simulink model "WaterDistSystem"  (R2023b)
settings: Solver=VariableStepAuto  StartTime=0.0  StopTime=inf  RelTol=1e-3
InitFcn:
  | seedGenerator
undefined symbols (not defined in the file or in its folder): hMin, maxCost, maxRep1, maxRep2, maxRep3, maxSteps, maxTime, meanFail1, meanFail2, meanFail3, minRep1, minRep2, minRep3, PenaltyCost, PenaltyPerformance, PenaltyResilience, PenaltySafety, RewardCost, RewardPerformance, RewardResilience, RewardSafety, rngSeed, singleReward, supCheck, supDeg, supFull, supNo, varFail1, varFail2, varFail3
libraries: simulink x4, rllib x1
settings Model: NumberOfSteps=10  SnapshotBufferSize=50  SnapshotInterval=50  Creator=sebru  LastModifiedBy=juliu
settings OptimizationCC: DefaultParameterBehavior=Inlined  EnhancedBackFolding=on  PassReuseOutputArgsAs=Individual arguments  ZeroExternalMemoryAtStartup=off  ZeroInternalMemoryAtStartup=off  OptimizeBlockOrder=speed  DifferentSizesBufferReuse=on  OptimizationCustomize=off  EfficientTunableParamExpr=on
settings DebuggingCC: AlgebraicLoopMsg=error  ParameterTunabilityLossMsg=error
settings ModelReferenceCC: EnableRefExpFcnMdlSchedulingChecks=on
settings SFSimCC: MATLABDynamicMemAlloc=off
settings RTWCC: Description=Embedded Coder  SystemTargetFile=ert.tlc  TemplateMakefile=ert_default_tmf
settings CodeAppCC: ForceParamTrailComments=on  IgnoreCustomStorageClasses=off  OperatorAnnotations=on  SimulinkDataObjDesc=on  SFDataObjDesc=on  InsertBlockDesc=on
settings ERTTargetCC: TargetLangStandard=C99 (ISO)  GenerateSampleERTMain=on  InlinedParameterPlacement=NonHierarchical  ERTCustomFileTemplate=example_file_process.tlc

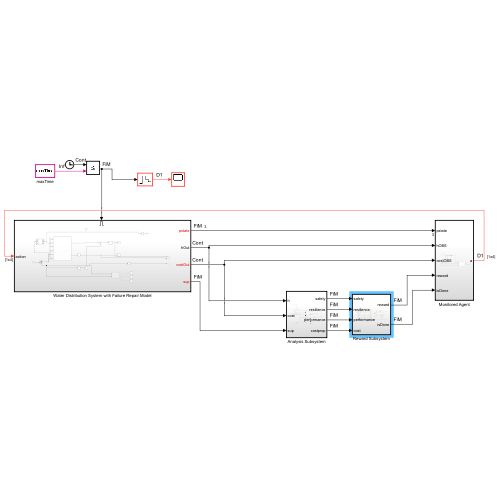
[thumbnail: Simulink's stored preview of the top-level diagram]
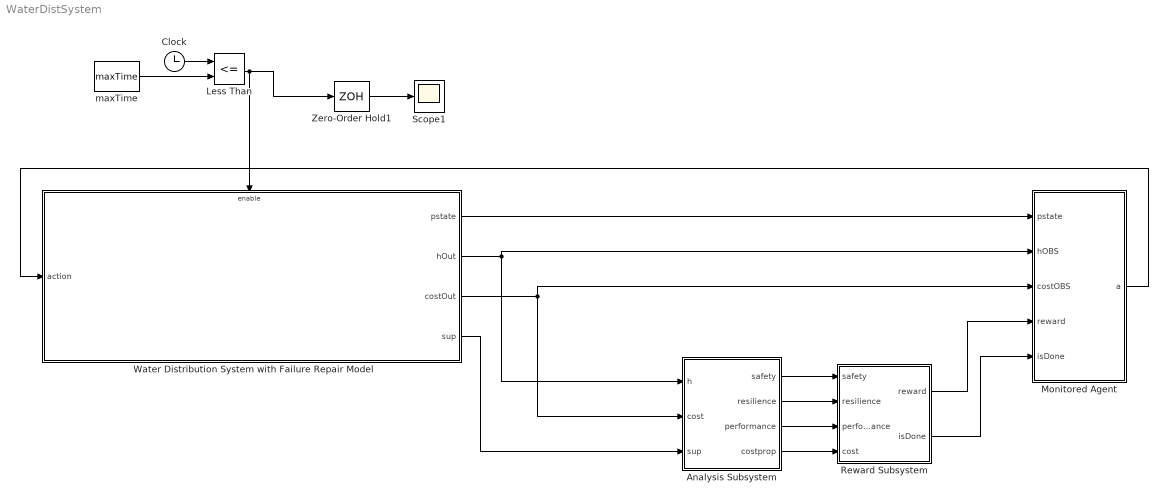
== system WaterDistSystem ==
  Analysis Subsystem : Subsystem
  Clock : Clock
  Less Than : RelationalOperator  Operator=<=  OutDataTypeStr=boolean  RndMeth=Simplest  InputSameDT=off
  Monitored Agent : Subsystem
  Reward Subsystem : Subsystem
  Scope1 : Scope
  Water Distribution System with Failure Repair Model : Subsystem  TreatAsAtomicUnit=on
      settings: MinAlgLoopOccurrences=on
  Zero-Order Hold1 : ZeroOrderHold  SampleTime=-1
  maxTime : Constant  Value=maxTime
  wires:
  Clock/1 -> Less Than/1
  Less Than/1 -> Zero-Order Hold1/1, Water Distribution System with Failure Repair Model/Enable
  maxTime/1 -> Less Than/2
  Monitored Agent/1(a) -> Water Distribution System with Failure Repair Model/1(action)
  Water Distribution System with Failure Repair Model/2(hOut) -> Analysis Subsystem/1(h), Monitored Agent/2(hOBS)
  Water Distribution System with Failure Repair Model/3(costOut) -> Analysis Subsystem/2(cost), Monitored Agent/3(costOBS)
  Water Distribution System with Failure Repair Model/1(pstate) -> Monitored Agent/1(pstate)
  Reward Subsystem/1(reward) -> Monitored Agent/4(reward)
  Reward Subsystem/2(isDone) -> Monitored Agent/5(isDone)
  Water Distribution System with Failure Repair Model/4(sup) -> Analysis Subsystem/3(sup)
  Zero-Order Hold1/1 -> Scope1/1
  Analysis Subsystem/2(resilience) -> Reward Subsystem/2(resilience)
  Analysis Subsystem/1(safety) -> Reward Subsystem/1(safety)
  Analysis Subsystem/4(costprop) -> Reward Subsystem/4(cost)
  Analysis Subsystem/3(performance) -> Reward Subsystem/3(performance)

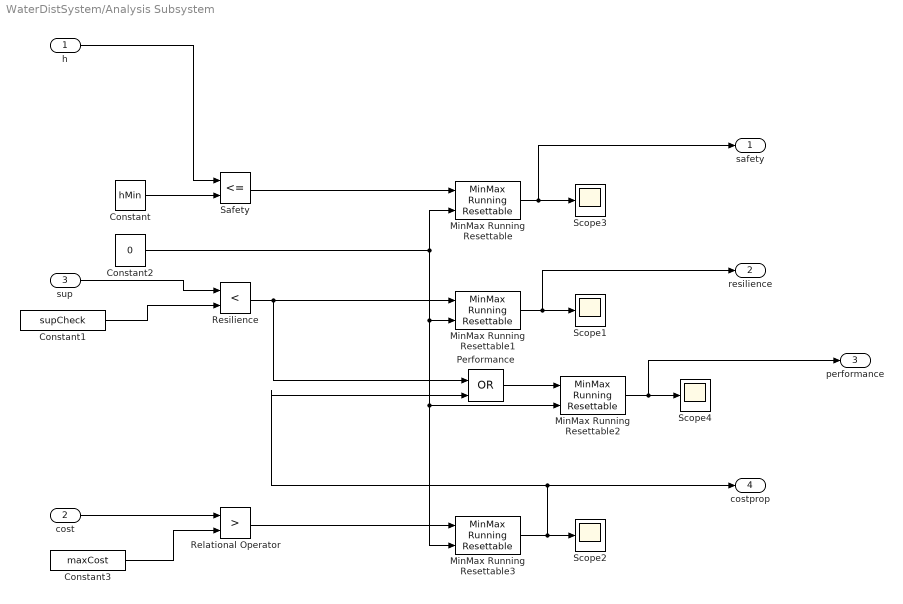
== system WaterDistSystem/Analysis Subsystem ==
  h : Inport
  cost : Inport  Port=2
  sup : Inport  Port=3
  Constant : Constant  Value=hMin
  Constant1 : Constant  Value=supCheck
  Constant2 : Constant  Value=0
  Constant3 : Constant  Value=maxCost
  MinMax Running Resettable{,1..3} (4 alike) : simulink/Math Operations/MinMax Running Resettable  Function=max  vinit=0.0
  Performance : Logic  Operator=OR  IconShape=distinctive  AllPortsSameDT=off  OutDataTypeStr=boolean
  Relational Operator : RelationalOperator  Operator=>  OutDataTypeStr=boolean  RndMeth=Simplest  InputSameDT=off
  Resilience : RelationalOperator  Operator=<  OutDataTypeStr=boolean  RndMeth=Floor  InputSameDT=off
  Safety : RelationalOperator  Operator=<=  OutDataTypeStr=boolean  RndMeth=Floor  InputSameDT=off
  Scope{1..4} (4 alike) : Scope
  safety : Outport
  resilience : Outport  Port=2
  performance : Outport  Port=3
  costprop : Outport  Port=4
  wires:
  Safety/1 -> MinMax Running Resettable/1
  Resilience/1 -> MinMax Running Resettable1/1, Performance/1
  Constant/1 -> Safety/2
  h/1 -> Safety/1
  MinMax Running Resettable2/1 -> performance/1, Scope4/1
  MinMax Running Resettable1/1 -> resilience/1, Scope1/1
  MinMax Running Resettable/1 -> safety/1, Scope3/1
  Performance/1 -> MinMax Running Resettable2/1
  Constant1/1 -> Resilience/2
  Constant2/1 -> MinMax Running Resettable/2, MinMax Running Resettable3/2, MinMax Running Resettable2/2, MinMax Running Resettable1/2
  Constant3/1 -> Relational Operator/2
  cost/1 -> Relational Operator/1
  Relational Operator/1 -> MinMax Running Resettable3/1
  MinMax Running Resettable3/1 -> Performance/2, costprop/1, Scope2/1
  sup/1 -> Resilience/1

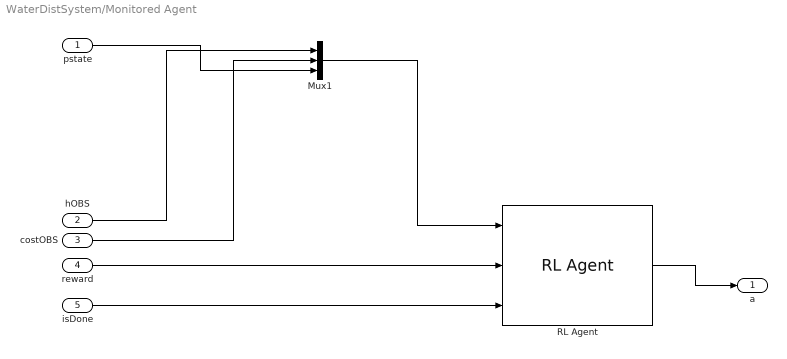
== system WaterDistSystem/Monitored Agent ==
  pstate : Inport
  hOBS : Inport  Port=2
  costOBS : Inport  Port=3
  reward : Inport  Port=4
  isDone : Inport  Port=5
  Mux1 : Mux  Inputs=3
  RL Agent : rllib/RL Agent  Agent=qAgent  ExternalActionAsInput=off  ProvideLastAction=off  ProvideCumRwd=off  TreatAsDirectFeedthrough=on  UseStrictObservationDataTypes=off
  a : Outport
  wires:
  Mux1/1 -> RL Agent/1
  hOBS/1 -> Mux1/1
  reward/1 -> RL Agent/2
  isDone/1 -> RL Agent/3
  RL Agent/1 -> a/1
  pstate/1 -> Mux1/3
  costOBS/1 -> Mux1/2

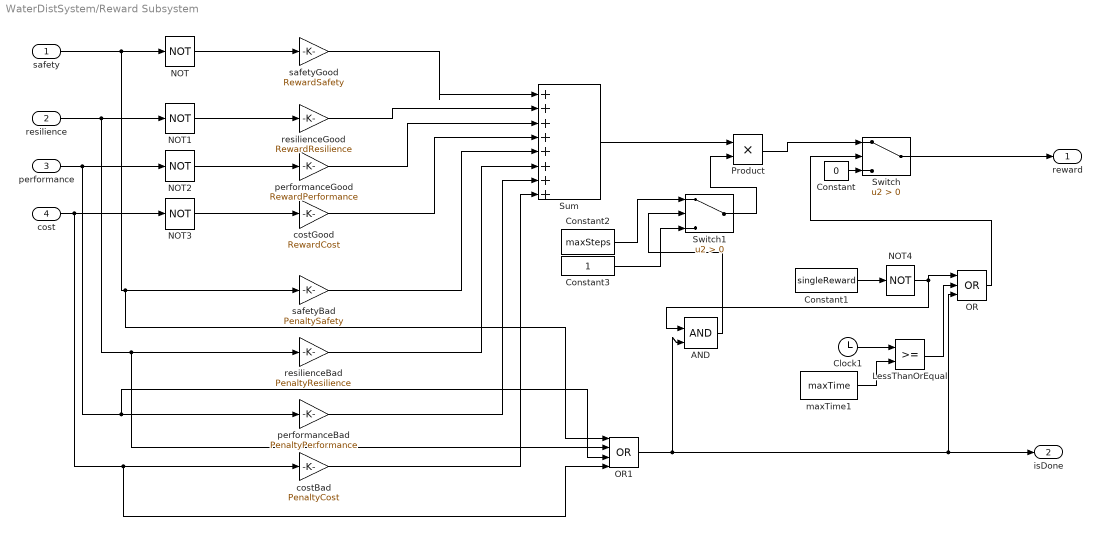
== system WaterDistSystem/Reward Subsystem ==
  safety : Inport
  resilience : Inport  Port=2
  performance : Inport  Port=3
  cost : Inport  Port=4
  AND : Logic  IconShape=distinctive  AllPortsSameDT=off  OutDataTypeStr=boolean
  Clock1 : Clock
  Constant : Constant  Value=0
  Constant1 : Constant  Value=singleReward
  Constant2 : Constant  Value=maxSteps
  Constant3 : Constant
  LessThanOrEqual : RelationalOperator  OutDataTypeStr=boolean  RndMeth=Simplest  InputSameDT=off
  NOT{,1..4} (5 alike) : Logic  Operator=NOT  IconShape=distinctive  AllPortsSameDT=off  OutDataTypeStr=boolean
  OR : Logic  Operator=OR  Inputs=3  IconShape=distinctive  AllPortsSameDT=off  OutDataTypeStr=boolean
  OR1 : Logic  Operator=OR  Inputs=4  IconShape=distinctive  AllPortsSameDT=off  OutDataTypeStr=boolean
  Product : Product
  Sum : Sum  Inputs=|++++++++
  Switch : Switch  Criteria=u2 > Threshold  SaturateOnIntegerOverflow=off  InputSameDT=off
  Switch1 : Switch  Criteria=u2 > Threshold  SaturateOnIntegerOverflow=off  InputSameDT=off
  costBad : Gain  Gain=PenaltyCost  OutDataTypeStr=double
  costGood : Gain  Gain=RewardCost  OutDataTypeStr=double
  maxTime1 : Constant  Value=maxTime
  performanceBad : Gain  Gain=PenaltyPerformance  OutDataTypeStr=double
  performanceGood : Gain  Gain=RewardPerformance  OutDataTypeStr=double
  resilienceBad : Gain  Gain=PenaltyResilience  OutDataTypeStr=double
  resilienceGood : Gain  Gain=RewardResilience  OutDataTypeStr=double
  safetyBad : Gain  Gain=PenaltySafety  OutDataTypeStr=double
  safetyGood : Gain  Gain=RewardSafety  OutDataTypeStr=double
  reward : Outport
  isDone : Outport  Port=2
  wires:
  NOT/1 -> safetyGood/1
  NOT1/1 -> resilienceGood/1
  NOT2/1 -> performanceGood/1
  performance/1 -> OR1/3, performanceBad/1, NOT2/1
  safety/1 -> OR1/1, safetyBad/1, NOT/1
  resilience/1 -> OR1/2, resilienceBad/1, NOT1/1
  safetyGood/1 -> Sum/1
  resilienceGood/1 -> Sum/2
  performanceGood/1 -> Sum/3
  safetyBad/1 -> Sum/5
  resilienceBad/1 -> Sum/6
  performanceBad/1 -> Sum/7
  NOT3/1 -> costGood/1
  cost/1 -> OR1/4, costBad/1, NOT3/1
  costGood/1 -> Sum/4
  costBad/1 -> Sum/8
  Constant/1 -> Switch/3
  Constant1/1 -> NOT4/1
  OR/1 -> Switch/2
  maxTime1/1 -> LessThanOrEqual/2
  NOT4/1 -> AND/1, OR/1
  Clock1/1 -> LessThanOrEqual/1
  LessThanOrEqual/1 -> OR/2
  Switch/1 -> reward/1
  Sum/1 -> Product/1
  Constant2/1 -> Switch1/1
  Constant3/1 -> Switch1/3
  OR1/1 -> AND/2, isDone/1, OR/3
  Product/1 -> Switch/1
  Switch1/1 -> Product/2
  AND/1 -> Switch1/2

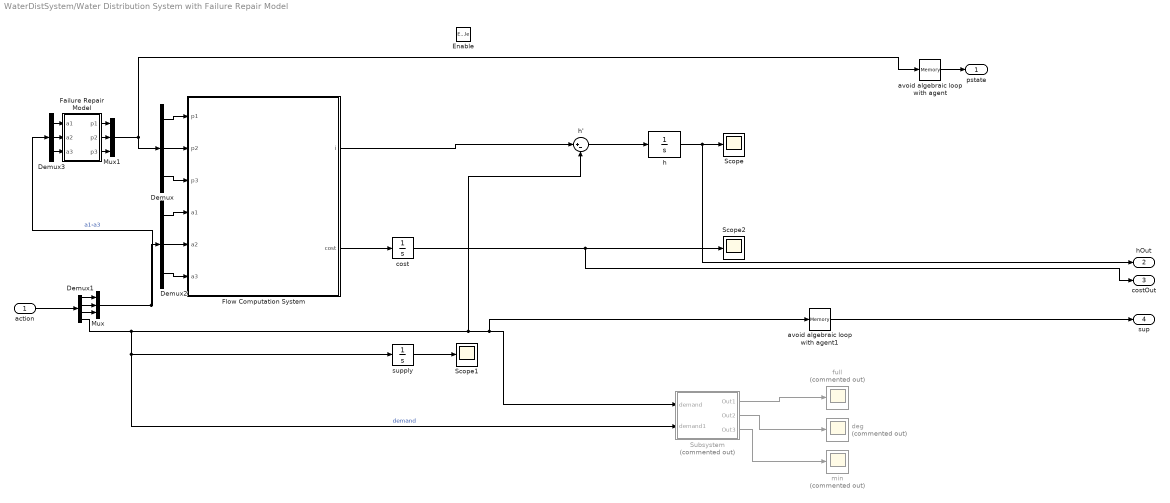
== system WaterDistSystem/Water Distribution System with Failure Repair Model ==
  action : Inport
  Enable : EnablePort
  Demux : Demux  Outputs=3
  Demux1 : Demux
  Demux2 : Demux  Outputs=3
  Demux3 : Demux  Outputs=3
  Failure Repair Model : Subsystem
  Flow Computation System : Subsystem  SystemSampleTime=0
  Mux : Mux  Inputs=3
  Mux1 : Mux  Inputs=3
  Scope : Scope
  Scope1 : Scope
  Scope2 : Scope
  Subsystem : Subsystem  Commented=on
  avoid algebraic loop with agent1 : Memory  InitialCondition=supFull
  avoid algebraic loop with agent : Memory
  cost : Integrator  LimitOutput=on  LowerSaturationLimit=0
  deg : Scope  Commented=on
  full : Scope  Commented=on
  h : Integrator  InitialCondition=5.5  LimitOutput=on  LowerSaturationLimit=0
  h' : Sum  Inputs=|+-
  min : Scope  Commented=on
  supply : Integrator  LimitOutput=on  LowerSaturationLimit=0
  pstate : Outport
  hOut : Outport  Port=2  InitialOutput=5.5
  costOut : Outport  Port=3  InitialOutput=0
  sup : Outport  Port=4  InitialOutput=0
  wires:
  Demux1/4 -> Subsystem/2(demand1), supply/1, Subsystem/1(demand), avoid algebraic loop with agent1/1, h'/2  "demand"
  h'/1 -> h/1
  cost/1 -> costOut/1, Scope2/1
  Flow Computation System/1(i) -> h'/1
  Flow Computation System/2(cost) -> cost/1
  h/1 -> hOut/1, Scope/1
  Demux/1 -> Flow Computation System/1(p1)
  Demux/2 -> Flow Computation System/2(p2)
  Demux/3 -> Flow Computation System/3(p3)
  action/1 -> Demux1/1
  Demux1/3 -> Mux/3
  Demux1/2 -> Mux/2
  Demux1/1 -> Mux/1
  Demux2/1 -> Flow Computation System/4(a1)
  Demux2/2 -> Flow Computation System/5(a2)
  Demux2/3 -> Flow Computation System/6(a3)
  Mux/1 -> Demux3/1, Demux2/1  "a1-a3"
  Demux3/1 -> Failure Repair Model/1(a1)
  Demux3/2 -> Failure Repair Model/2(a2)
  Demux3/3 -> Failure Repair Model/3(a3)
  Failure Repair Model/2(p2) -> Mux1/2
  Failure Repair Model/3(p3) -> Mux1/3
  Failure Repair Model/1(p1) -> Mux1/1
  avoid algebraic loop with agent/1 -> pstate/1
  Mux1/1 -> avoid algebraic loop with agent/1, Demux/1
  supply/1 -> Scope1/1
  avoid algebraic loop with agent1/1 -> sup/1
  Subsystem/2(Out2) -> deg/1
  Subsystem/3(Out3) -> min/1
  Subsystem/1(Out1) -> full/1

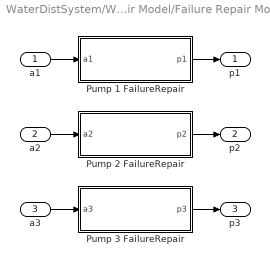
== system WaterDistSystem/Water Distribution System with Failure Repair Model/Failure Repair Model ==
  a1 : Inport
  a2 : Inport  Port=2
  a3 : Inport  Port=3
  Pump 1 FailureRepair : Subsystem  TreatAsAtomicUnit=on  SystemSampleTime=0
  Pump 2 FailureRepair : Subsystem  TreatAsAtomicUnit=on  SystemSampleTime=0
  Pump 3 FailureRepair : Subsystem  TreatAsAtomicUnit=on  SystemSampleTime=0
  p1 : Outport
  p2 : Outport  Port=2
  p3 : Outport  Port=3
  wires:
  Pump 2 FailureRepair/1(p2) -> p2/1
  a3/1 -> Pump 3 FailureRepair/1(a3)
  Pump 1 FailureRepair/1(p1) -> p1/1
  Pump 3 FailureRepair/1(p3) -> p3/1
  a2/1 -> Pump 2 FailureRepair/1(a2)
  a1/1 -> Pump 1 FailureRepair/1(a1)

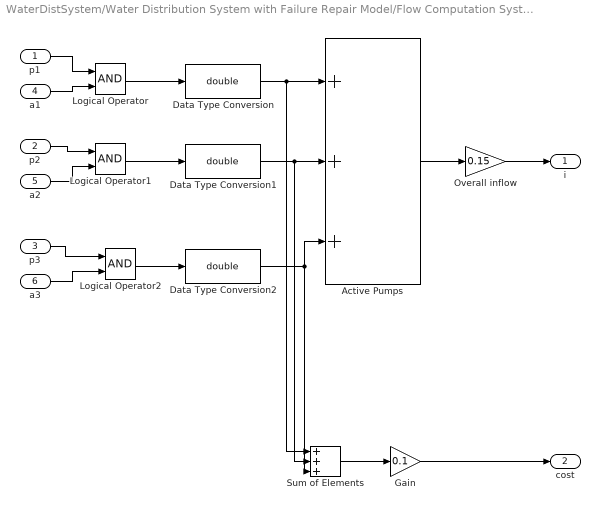
== system WaterDistSystem/Water Distribution System with Failure Repair Model/Flow Computation System ==
  p1 : Inport
  p2 : Inport  Port=2
  p3 : Inport  Port=3
  a1 : Inport  Port=4
  a2 : Inport  Port=5
  a3 : Inport  Port=6
  Active Pumps : Sum  Inputs=+++
  Data Type Conversion : DataTypeConversion  OutDataTypeStr=double  SaturateOnIntegerOverflow=off  RndMeth=Floor
  Data Type Conversion1 : DataTypeConversion  OutDataTypeStr=double  SaturateOnIntegerOverflow=off  RndMeth=Floor
  Data Type Conversion2 : DataTypeConversion  OutDataTypeStr=double  SaturateOnIntegerOverflow=off  RndMeth=Floor
  Gain : Gain  Gain=0.1
  Logical Operator : Logic  AllPortsSameDT=off  OutDataTypeStr=boolean
  Logical Operator1 : Logic  AllPortsSameDT=off  OutDataTypeStr=boolean
  Logical Operator2 : Logic  AllPortsSameDT=off  OutDataTypeStr=boolean
  Overall inflow : Gain  Gain=0.15
  Sum of Elements : Sum  Inputs=+++
  i : Outport
  cost : Outport  Port=2
  wires:
  a1/1 -> Logical Operator/2
  a2/1 -> Logical Operator1/2
  a3/1 -> Logical Operator2/2
  Active Pumps/1 -> Overall inflow/1
  Logical Operator1/1 -> Data Type Conversion1/1
  Logical Operator2/1 -> Data Type Conversion2/1
  Logical Operator/1 -> Data Type Conversion/1
  Data Type Conversion/1 -> Sum of Elements/1, Active Pumps/1
  Data Type Conversion1/1 -> Sum of Elements/2, Active Pumps/2
  Data Type Conversion2/1 -> Sum of Elements/3, Active Pumps/3
  Overall inflow/1 -> i/1
  p1/1 -> Logical Operator/1
  p2/1 -> Logical Operator1/1
  p3/1 -> Logical Operator2/1
  Sum of Elements/1 -> Gain/1
  Gain/1 -> cost/1

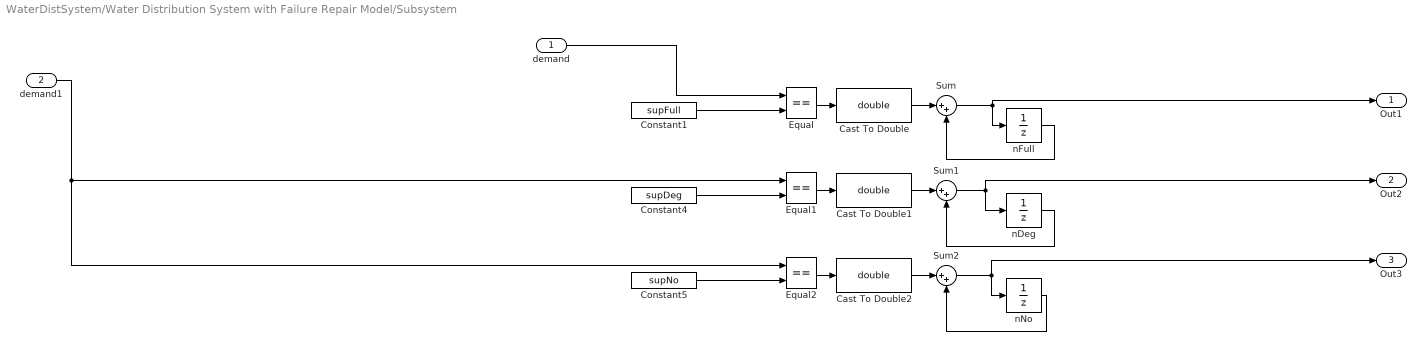
== system WaterDistSystem/Water Distribution System with Failure Repair Model/Subsystem ==
  demand : Inport
  demand1 : Inport  Port=2
  Cast To Double : DataTypeConversion  OutDataTypeStr=double  SaturateOnIntegerOverflow=off  RndMeth=Floor
  Cast To Double1 : DataTypeConversion  OutDataTypeStr=double  SaturateOnIntegerOverflow=off  RndMeth=Floor
  Cast To Double2 : DataTypeConversion  OutDataTypeStr=double  SaturateOnIntegerOverflow=off  RndMeth=Floor
  Constant1 : Constant  Value=supFull
  Constant4 : Constant  Value=supDeg
  Constant5 : Constant  Value=supNo
  Equal : RelationalOperator  Operator===  OutDataTypeStr=boolean  RndMeth=Simplest  InputSameDT=off
  Equal1 : RelationalOperator  Operator===  OutDataTypeStr=boolean  RndMeth=Simplest  InputSameDT=off
  Equal2 : RelationalOperator  Operator===  OutDataTypeStr=boolean  RndMeth=Simplest  InputSameDT=off
  Sum : Sum  Inputs=|++
  Sum1 : Sum  Inputs=|++
  Sum2 : Sum  Inputs=|++
  nDeg : UnitDelay  HasFrameUpgradeWarning=on
  nFull : UnitDelay  HasFrameUpgradeWarning=on
  nNo : UnitDelay  HasFrameUpgradeWarning=on
  Out1 : Outport
  Out2 : Outport  Port=2
  Out3 : Outport  Port=3
  wires:
  nDeg/1 -> Sum1/2
  nNo/1 -> Sum2/2
  Cast To Double/1 -> Sum/1
  Equal/1 -> Cast To Double/1
  Equal1/1 -> Cast To Double1/1
  Sum1/1 -> Out2/1, nDeg/1
  Equal2/1 -> Cast To Double2/1
  Sum/1 -> Out1/1, nFull/1
  Cast To Double1/1 -> Sum1/1
  demand1/1 -> Equal2/1, Equal1/1
  Constant1/1 -> Equal/2
  nFull/1 -> Sum/2
  Constant4/1 -> Equal1/2
  Sum2/1 -> Out3/1, nNo/1
  Constant5/1 -> Equal2/2
  Cast To Double2/1 -> Sum2/1
  demand/1 -> Equal/1

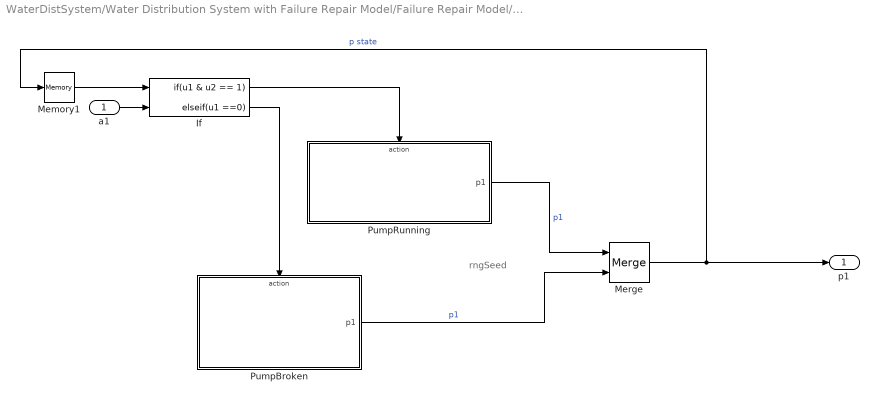
== system WaterDistSystem/Water Distribution System with Failure Repair Model/Failure Repair Model/Pump 1 FailureRepair ==
  note: rngSeed
  a1 : Inport
  If : If  NumInputs=2  IfExpression=u1 & u2 == 1  ElseIfExpressions=u1 ==0  ShowElse=off
  Memory1 : Memory  InitialCondition=1
  Merge : Merge  InitialOutput=1
  PumpBroken : Subsystem  TreatAsAtomicUnit=on
  PumpRunning : Subsystem  TreatAsAtomicUnit=on
  p1 : Outport
  wires:
  If/2 -> PumpBroken/Action
  If/1 -> PumpRunning/Action
  a1/1 -> If/2
  PumpRunning/1(p1) -> Merge/1  "p1"
  PumpBroken/1(p1) -> Merge/2  "p1"
  Merge/1 -> p1/1, Memory1/1  "p state"
  Memory1/1 -> If/1

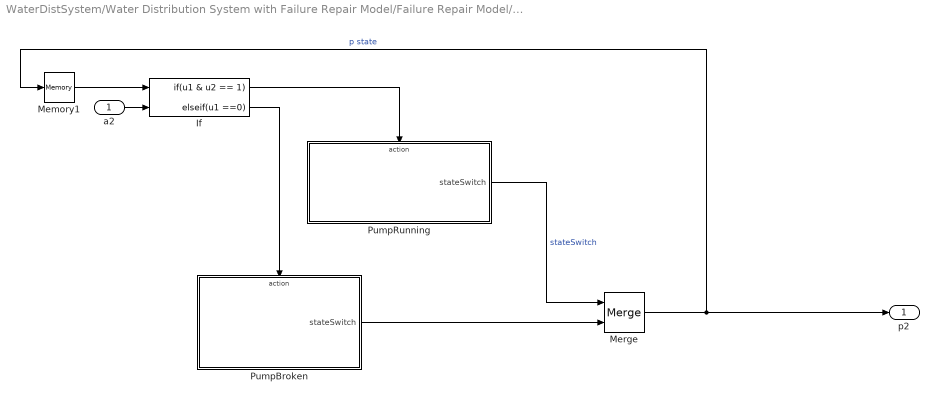
== system WaterDistSystem/Water Distribution System with Failure Repair Model/Failure Repair Model/Pump 2 FailureRepair ==
  a2 : Inport
  If : If  NumInputs=2  IfExpression=u1 & u2 == 1  ElseIfExpressions=u1 ==0  ShowElse=off
  Memory1 : Memory  InitialCondition=1
  Merge : Merge  InitialOutput=1
  PumpBroken : Subsystem  TreatAsAtomicUnit=on
  PumpRunning : Subsystem  TreatAsAtomicUnit=on
  p2 : Outport
  wires:
  If/2 -> PumpBroken/Action
  If/1 -> PumpRunning/Action
  a2/1 -> If/2
  PumpRunning/1(stateSwitch) -> Merge/1  "stateSwitch"
  PumpBroken/1(stateSwitch) -> Merge/2
  Merge/1 -> Memory1/1, p2/1  "p state"
  Memory1/1 -> If/1

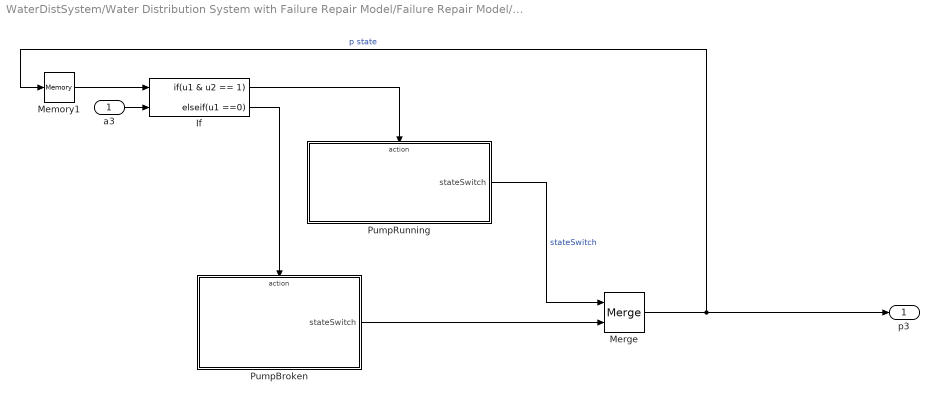
== system WaterDistSystem/Water Distribution System with Failure Repair Model/Failure Repair Model/Pump 3 FailureRepair ==
  a3 : Inport
  If : If  NumInputs=2  IfExpression=u1 & u2 == 1  ElseIfExpressions=u1 ==0  ShowElse=off
  Memory1 : Memory  InitialCondition=1
  Merge : Merge  InitialOutput=1
  PumpBroken : Subsystem  TreatAsAtomicUnit=on
  PumpRunning : Subsystem  TreatAsAtomicUnit=on
  p3 : Outport
  wires:
  If/2 -> PumpBroken/Action
  If/1 -> PumpRunning/Action
  a3/1 -> If/2
  PumpRunning/1(stateSwitch) -> Merge/1  "stateSwitch"
  PumpBroken/1(stateSwitch) -> Merge/2
  Merge/1 -> Memory1/1, p3/1  "p state"
  Memory1/1 -> If/1

== system WaterDistSystem/Water Distribution System with Failure Repair Model/Failure Repair Model/Pump 1 FailureRepair/PumpBroken ==
  Action Port : ActionPort  ActionPortLabel=elseif(u1 ==0)
  Memory : Memory
  Resettable Subsystem : Subsystem  TreatAsAtomicUnit=on
  p1 : Outport
  wires:
  Resettable Subsystem/1(p1) -> Memory/1, p1/1
  Memory/1 -> Resettable Subsystem/Reset  "memp1"

== system WaterDistSystem/Water Distribution System with Failure Repair Model/Failure Repair Model/Pump 1 FailureRepair/PumpRunning ==
  Action Port : ActionPort  ActionPortLabel=if(u1 & u2 == 1)
  Memory2 : Memory  InheritSampleTime=on
  NOT : Logic  Operator=NOT  IconShape=distinctive  AllPortsSameDT=off  OutDataTypeStr=boolean
  Resettable Subsystem : Subsystem  Priority=2  TreatAsAtomicUnit=on
  p1 : Outport
  wires:
  Resettable Subsystem/1(Output1) -> NOT/1, p1/1
  NOT/1 -> Memory2/1
  Memory2/1 -> Resettable Subsystem/Reset  "memp1"

== system WaterDistSystem/Water Distribution System with Failure Repair Model/Failure Repair Model/Pump 2 FailureRepair/PumpBroken ==
  Action Port : ActionPort  ActionPortLabel=elseif(u1 ==0)
  Memory : Memory
  Resettable Subsystem : Subsystem  TreatAsAtomicUnit=on
  stateSwitch : Outport
  wires:
  Resettable Subsystem/1(stateSwitch) -> Memory/1, stateSwitch/1
  Memory/1 -> Resettable Subsystem/Reset  "memp1"

== system WaterDistSystem/Water Distribution System with Failure Repair Model/Failure Repair Model/Pump 2 FailureRepair/PumpRunning ==
  Action Port : ActionPort  ActionPortLabel=if(u1 & u2 == 1)
  Memory2 : Memory  InheritSampleTime=on
  NOT : Logic  Operator=NOT  IconShape=distinctive  AllPortsSameDT=off  OutDataTypeStr=boolean
  Resettable Subsystem : Subsystem  Priority=2  TreatAsAtomicUnit=on
  stateSwitch : Outport
  wires:
  Resettable Subsystem/1(Output1) -> NOT/1, stateSwitch/1  "memp1"
  NOT/1 -> Memory2/1
  Memory2/1 -> Resettable Subsystem/Reset  "memp1"

== system WaterDistSystem/Water Distribution System with Failure Repair Model/Failure Repair Model/Pump 3 FailureRepair/PumpBroken ==
  Action Port : ActionPort  ActionPortLabel=elseif(u1 ==0)
  Memory : Memory
  Resettable Subsystem : Subsystem  TreatAsAtomicUnit=on
  stateSwitch : Outport
  wires:
  Resettable Subsystem/1(stateSwitch) -> Memory/1, stateSwitch/1
  Memory/1 -> Resettable Subsystem/Reset  "memp1"

== system WaterDistSystem/Water Distribution System with Failure Repair Model/Failure Repair Model/Pump 3 FailureRepair/PumpRunning ==
  Action Port : ActionPort  ActionPortLabel=if(u1 & u2 == 1)
  Memory2 : Memory  InheritSampleTime=on
  NOT : Logic  Operator=NOT  IconShape=distinctive  AllPortsSameDT=off  OutDataTypeStr=boolean
  Resettable Subsystem : Subsystem  Priority=2  TreatAsAtomicUnit=on
  stateSwitch : Outport
  wires:
  Resettable Subsystem/1(Output1) -> NOT/1, stateSwitch/1  "memp1"
  NOT/1 -> Memory2/1
  Memory2/1 -> Resettable Subsystem/Reset  "memp1"

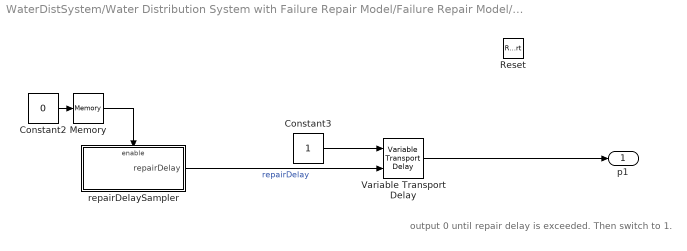
== system WaterDistSystem/Water Distribution System with Failure Repair Model/Failure Repair Model/Pump 1 FailureRepair/PumpBroken/Resettable Subsystem ==
  note: output 0 until repair delay is exceeded. Then switch to 1.
  Reset : ResetPort  DisableCoverage=on
  Constant2 : Constant  Value=0
  Constant3 : Constant
  Memory : Memory  InitialCondition=1
  Variable Transport Delay : VariableTransportDelay  VariableDelayType=Variable transport delay  MaximumDelay=100
  repairDelaySampler : Subsystem  TreatAsAtomicUnit=on
  p1 : Outport
  wires:
  Constant2/1 -> Memory/1
  Memory/1 -> repairDelaySampler/Enable
  repairDelaySampler/1(repairDelay) -> Variable Transport Delay/2  "repairDelay"
  Variable Transport Delay/1 -> p1/1
  Constant3/1 -> Variable Transport Delay/1

== system WaterDistSystem/Water Distribution System with Failure Repair Model/Failure Repair Model/Pump 1 FailureRepair/PumpRunning/Resettable Subsystem ==
  note: output 1 until failure delay is exceeded. Then switch to 0.
  note: integrates time
  Reset : ResetPort  DisableCoverage=on
  Constant2 : Constant  Value=0
  Constant3 : Constant  Value=0
  FailureDelaySampler : Subsystem  TreatAsAtomicUnit=on
  Memory : Memory  InitialCondition=1
  Variable Transport Delay : VariableTransportDelay  VariableDelayType=Variable transport delay  MaximumDelay=100  InitialOutput=1
  Output1 : Outport
  wires:
  Constant2/1 -> Memory/1
  Memory/1 -> FailureDelaySampler/Enable
  Variable Transport Delay/1 -> Output1/1
  Constant3/1 -> Variable Transport Delay/1
  FailureDelaySampler/1(Input) -> Variable Transport Delay/2  "failureDelay"

== system WaterDistSystem/Water Distribution System with Failure Repair Model/Failure Repair Model/Pump 2 FailureRepair/PumpBroken/Resettable Subsystem ==
  note: output 0 until repair delay is exceeded. Then switch to 1.
  Reset : ResetPort  DisableCoverage=on
  Constant2 : Constant  Value=0
  Constant3 : Constant
  Memory : Memory  InitialCondition=1
  Variable Transport Delay : VariableTransportDelay  VariableDelayType=Variable transport delay  MaximumDelay=100
  repairDelaySampler : Subsystem  TreatAsAtomicUnit=on
  stateSwitch : Outport
  wires:
  Variable Transport Delay/1 -> stateSwitch/1
  repairDelaySampler/1(repairDelay) -> Variable Transport Delay/2  "failureDelay"
  Constant2/1 -> Memory/1
  Memory/1 -> repairDelaySampler/Enable
  Constant3/1 -> Variable Transport Delay/1

== system WaterDistSystem/Water Distribution System with Failure Repair Model/Failure Repair Model/Pump 2 FailureRepair/PumpRunning/Resettable Subsystem ==
  note: output 1 until failure delay is exceeded. Then switch to 0.
  note: integrates time
  Reset : ResetPort  DisableCoverage=on
  Constant2 : Constant  Value=0
  Constant3 : Constant  Value=0
  FailureDelaySampler : Subsystem  TreatAsAtomicUnit=on
  Memory : Memory  InitialCondition=1
  Variable Transport Delay : VariableTransportDelay  VariableDelayType=Variable transport delay  MaximumDelay=100  InitialOutput=1
  Output1 : Outport
  wires:
  FailureDelaySampler/1(Input) -> Variable Transport Delay/2  "breakdelay"
  Constant2/1 -> Memory/1
  Memory/1 -> FailureDelaySampler/Enable
  Variable Transport Delay/1 -> Output1/1
  Constant3/1 -> Variable Transport Delay/1

== system WaterDistSystem/Water Distribution System with Failure Repair Model/Failure Repair Model/Pump 3 FailureRepair/PumpBroken/Resettable Subsystem ==
  note: output 0 until repair delay is exceeded. Then switch to 1.
  Reset : ResetPort  DisableCoverage=on
  Constant2 : Constant  Value=0
  Constant3 : Constant
  Memory : Memory  InitialCondition=1
  Variable Transport Delay : VariableTransportDelay  VariableDelayType=Variable transport delay  MaximumDelay=100
  repairDelaySampler : Subsystem  TreatAsAtomicUnit=on
  stateSwitch : Outport
  wires:
  Variable Transport Delay/1 -> stateSwitch/1
  Constant2/1 -> Memory/1
  Memory/1 -> repairDelaySampler/Enable
  Constant3/1 -> Variable Transport Delay/1
  repairDelaySampler/1(repairDelay) -> Variable Transport Delay/2  "failureDelay"

== system WaterDistSystem/Water Distribution System with Failure Repair Model/Failure Repair Model/Pump 3 FailureRepair/PumpRunning/Resettable Subsystem ==
  note: output 1 until failure delay is exceeded. Then switch to 0.
  note: integrates time
  Reset : ResetPort  DisableCoverage=on
  Constant2 : Constant  Value=0
  Constant3 : Constant  Value=0
  FailureDelaySampler : Subsystem  TreatAsAtomicUnit=on
  Memory : Memory  InitialCondition=1
  Variable Transport Delay : VariableTransportDelay  VariableDelayType=Variable transport delay  MaximumDelay=100  InitialOutput=1
  Output1 : Outport
  wires:
  FailureDelaySampler/1(Input) -> Variable Transport Delay/2  "breakdelay"
  Constant2/1 -> Memory/1
  Memory/1 -> FailureDelaySampler/Enable
  Variable Transport Delay/1 -> Output1/1
  Constant3/1 -> Variable Transport Delay/1

== system WaterDistSystem/Water Distribution System with Failure Repair Model/Failure Repair Model/Pump 1 FailureRepair/PumpBroken/Resettable Subsystem/repairDelaySampler ==
  Enable : EnablePort
  Uniform Random Number : UniformRandomNumber  Minimum=minRep1  Maximum=maxRep1  Seed=rngSeed  SampleTime=0
  repairDelay : Outport
  wires:
  Uniform Random Number/1 -> repairDelay/1

== system WaterDistSystem/Water Distribution System with Failure Repair Model/Failure Repair Model/Pump 1 FailureRepair/PumpRunning/Resettable Subsystem/FailureDelaySampler ==
  Enable : EnablePort
  Abs : Abs  SaturateOnIntegerOverflow=off
  Random Number : RandomNumber  Mean=meanFail1  Variance=varFail1  Seed=rngSeed  SampleTime=0
  Input : Outport
  wires:
  Random Number/1 -> Abs/1
  Abs/1 -> Input/1

== system WaterDistSystem/Water Distribution System with Failure Repair Model/Failure Repair Model/Pump 2 FailureRepair/PumpBroken/Resettable Subsystem/repairDelaySampler ==
  Enable : EnablePort
  Uniform Random Number : UniformRandomNumber  Minimum=minRep2  Maximum=maxRep2  Seed=rngSeed  SampleTime=0
  repairDelay : Outport
  wires:
  Uniform Random Number/1 -> repairDelay/1

== system WaterDistSystem/Water Distribution System with Failure Repair Model/Failure Repair Model/Pump 2 FailureRepair/PumpRunning/Resettable Subsystem/FailureDelaySampler ==
  Enable : EnablePort
  Abs : Abs  SaturateOnIntegerOverflow=off
  Random Number : RandomNumber  Mean=meanFail2  Variance=varFail2  Seed=rngSeed  SampleTime=0
  Input : Outport
  wires:
  Random Number/1 -> Abs/1
  Abs/1 -> Input/1

== system WaterDistSystem/Water Distribution System with Failure Repair Model/Failure Repair Model/Pump 3 FailureRepair/PumpBroken/Resettable Subsystem/repairDelaySampler ==
  Enable : EnablePort
  Uniform Random Number : UniformRandomNumber  Minimum=minRep3  Maximum=maxRep3  Seed=rngSeed  SampleTime=0
  repairDelay : Outport
  wires:
  Uniform Random Number/1 -> repairDelay/1

== system WaterDistSystem/Water Distribution System with Failure Repair Model/Failure Repair Model/Pump 3 FailureRepair/PumpRunning/Resettable Subsystem/FailureDelaySampler ==
  Enable : EnablePort
  Abs : Abs  SaturateOnIntegerOverflow=off
  Random Number : RandomNumber  Mean=meanFail3  Variance=varFail3  Seed=rngSeed  SampleTime=0
  Input : Outport
  wires:
  Random Number/1 -> Abs/1
  Abs/1 -> Input/1
